simulink library "NFSModelsLibrary"  (R2020a)
settings: Solver=VariableStepAuto  StartTime=0.0  StopTime=10.0  RelTol=1e-3
undefined symbols (not defined in the file or in its folder): Earth, F, Light, MIL, Newton, nfs, Raphson, sigbuilder_block, WGS84
libraries: sharedutil x3, simulink x2, ModelsLibrary x2, $bdroot x2, aerolibwind2 x2, aerolibtransform2 x1
(part 2 of 3)

== system NFSModelsLibrary/3-AxisRateGyro/Noise Check/No Noise ==
  In : Inport
  Gain : Gain  Gain=0
  "Out " : Outport  VectorParamsAs1DForOutWhenUnconnected=off
  wires:
  Gain/1 -> "Out "/1
  In/1 -> Gain/1

== system NFSModelsLibrary/3-AxisRateGyro/Noise Check/Noisy Signal ==
  In : Inport
  "Out " : Outport  VectorParamsAs1DForOutWhenUnconnected=off
  wires:
  In/1 -> "Out "/1

== system NFSModelsLibrary/Aerodynamic Forces and Moments Derivatives/Forces/Aerodynamic Forces ==
  note: Since the forces and moments are in stability axis,
      | the beta has been multiplied with zero.
  CL : Inport  PortDimensions=1
  CD : Inport  Port=2  PortDimensions=1
  CY : Inport  Port=3  PortDimensions=1
  Dynamic Pressure : Inport  Port=4  PortDimensions=1
  Alpha : Inport  Port=5  PortDimensions=1
  Beta : Inport  Port=6  PortDimensions=1
  ChSign : Gain  Gain=-1  SaturateOnIntegerOverflow=on  OutDataTypeStr=Inherit: Same as input  ParamDataTypeStr=Inherit: Same as input
  ChSign1 : Gain  Gain=-1  SaturateOnIntegerOverflow=on  OutDataTypeStr=Inherit: Same as input  ParamDataTypeStr=Inherit: Same as input
  ChSign2 : Gain  Gain=0  SaturateOnIntegerOverflow=on  OutDataTypeStr=Inherit: Same as input  ParamDataTypeStr=Inherit: Same as input
  Mux : Mux  Inputs=3
  Product{,2..4} (4 alike) : Product  InputSameDT=on  SaturateOnIntegerOverflow=on  OutDataTypeStr=Inherit: Same as first input
  Product1 : Product  Multiplication=Matrix(*)  InputSameDT=on  SaturateOnIntegerOverflow=on  OutDataTypeStr=Inherit: Same as first input
  Wind2Body TM : Subsystem
  Wing Area : Constant  Value=nfs.refarea
  Aerodynamic Forces : Outport  PortDimensions=[3,1]  VectorParamsAs1DForOutWhenUnconnected=off
  wires:
  ChSign2/1 -> Wind2Body TM/2(Beta)
  Mux/1 -> Product1/2
  Product4/1 -> Mux/3
  Product3/1 -> Mux/2
  Product2/1 -> Mux/1
  ChSign1/1 -> Product4/2
  CY/1 -> Product3/2
  ChSign/1 -> Product2/2
  Product/1 -> Product4/1, Product3/1, Product2/1
  Wing Area/1 -> Product/2
  Dynamic Pressure/1 -> Product/1
  Alpha/1 -> Wind2Body TM/1(Alpha)
  CL/1 -> ChSign1/1
  CD/1 -> ChSign/1
  Beta/1 -> ChSign2/1
  Product1/1 -> Aerodynamic Forces/1
  Wind2Body TM/1(T_BW) -> Product1/1

== system NFSModelsLibrary/Aerodynamic Forces and Moments Derivatives/Forces/Force Coefficients Calculator ==
  Linear Velocity : Inport  PortDimensions=[3,1]
  Alpha : Inport  Port=2  PortDimensions=1
  Beta : Inport  Port=3
  Angular Velocity : Inport  Port=4  PortDimensions=[3,1]
  Control : Inport  Port=5  PortDimensions=[4,1]
  Alphadot : Inport  Port=6  PortDimensions=1
  Mach : Inport  Port=7
  Alpha2 : InportShadow  Port=2  PortDimensions=1
  Angular Velocity1 : InportShadow  Port=4  PortDimensions=[3,1]
  Control1 : InportShadow  Port=5  PortDimensions=[4,1]
  Demux1 : Demux  Outputs=3
      settings: DisplayOption=none
  Demux2 : Demux  Outputs=3
      settings: DisplayOption=none
  Demux3 : Demux
      settings: DisplayOption=none
  Demux4 : Demux
      settings: DisplayOption=none
  Drag Coefficient : Subsystem  mask{cD0=nfs.aero.cD0}
  Lift Coefficient : Subsystem  mask{cL0=nfs.aero.cL0, meanchord=nfs.meanchord}
      mask prompts: meanchord "Mean Aerodynamic Chord"
  Linear Velocity1 : InportShadow  PortDimensions=[3,1]
  Mach1 : InportShadow  Port=7
  SideForce Coefficient : Subsystem
  Terminator{,1..4} (5 alike) : Terminator
  CL : Outport  VectorParamsAs1DForOutWhenUnconnected=off
  CD : Outport  Port=2  VectorParamsAs1DForOutWhenUnconnected=off
  CY : Outport  Port=3  VectorParamsAs1DForOutWhenUnconnected=off
  wires:
  Linear Velocity1/1 -> SideForce Coefficient/1(Linear Velocity)
  Demux3/2 -> Lift Coefficient/4(DeltaFlap)
  Mach1/1 -> Drag Coefficient/7(Mach)
  Demux4/1 -> Drag Coefficient/3(DeltaElevator)
  Demux4/3 -> Drag Coefficient/5(DeltaAileron), SideForce Coefficient/5(DeltaAileron)
  Demux4/4 -> Drag Coefficient/6(DeltaRudder), SideForce Coefficient/6(DeltaRudder)
  Demux2/2 -> Terminator2/1
  Alpha/1 -> Lift Coefficient/2(Alpha)
  Demux3/3 -> Terminator3/1
  Demux3/4 -> Terminator4/1
  Demux1/2 -> Lift Coefficient/6(Q)
  Mach/1 -> Lift Coefficient/7(Mach)
  Demux4/2 -> Drag Coefficient/4(DeltaFlap)
  Angular Velocity/1 -> Demux1/1
  Control/1 -> Demux3/1
  Demux1/1 -> Terminator/1
  Beta/1 -> SideForce Coefficient/2(Beta)
  Angular Velocity1/1 -> Demux2/1
  Demux2/3 -> SideForce Coefficient/4(R)
  Control1/1 -> Demux4/1
  Demux3/1 -> Lift Coefficient/3(DeltaElevator)
  Demux2/1 -> SideForce Coefficient/3(P)
  Lift Coefficient/1(CL) -> Drag Coefficient/1(CL), CL/1
  Alphadot/1 -> Lift Coefficient/5(Alphadot)
  Demux1/3 -> Terminator1/1
  Alpha2/1 -> Drag Coefficient/2(alpha)
  Drag Coefficient/1(CD) -> CD/1
  SideForce Coefficient/1(CY) -> CY/1
  Linear Velocity/1 -> Lift Coefficient/1(Linear Velocity)

== system NFSModelsLibrary/Aerodynamic Forces and Moments Derivatives/Moments/Aerodynamic Moment  ==
  note: Since the forces and moments are in stability axis,
      | the beta has been multiplied with zero.
  Cl : Inport
  Cm : Inport  Port=2
  Cn : Inport  Port=3
  Dynamic Pressure : Inport  Port=4
  Alpha : Inport  Port=5  PortDimensions=1
  Beta : Inport  Port=6  PortDimensions=1
  Dynamic Pressure1 : InportShadow  Port=4
  Dynamic Pressure2 : InportShadow  Port=4
  Gain : Gain  Gain=0
  Mux : Mux  Inputs=3
  Pitch : Product  Inputs=4  InputSameDT=on  SaturateOnIntegerOverflow=on  OutDataTypeStr=Inherit: Same as first input
  Product1 : Product  Multiplication=Matrix(*)  InputSameDT=on  SaturateOnIntegerOverflow=on  OutDataTypeStr=Inherit: Same as first input
  Roll : Product  Inputs=4  InputSameDT=on  SaturateOnIntegerOverflow=on  OutDataTypeStr=Inherit: Same as first input
  Wind2Body TM : Subsystem
  Wing area : Constant  Value=nfs.refarea
  Wing chord : Constant  Value=nfs.meanchord
  Wing span : Constant  Value=nfs.span
  Wing span2 : Constant  Value=nfs.span
  Yaw : Product  Inputs=4  InputSameDT=on  SaturateOnIntegerOverflow=on  OutDataTypeStr=Inherit: Same as first input
  Aerodynamic Moments : Outport  PortDimensions=[3,1]  VectorParamsAs1DForOutWhenUnconnected=off
  wires:
  Gain/1 -> Wind2Body TM/2(Beta)
  Product1/1 -> Aerodynamic Moments/1
  Mux/1 -> Product1/2
  Alpha/1 -> Wind2Body TM/1(Alpha)
  Beta/1 -> Gain/1
  Wind2Body TM/1(T_BW) -> Product1/1
  Wing span/1 -> Roll/3
  Wing chord/1 -> Pitch/3
  Dynamic Pressure/1 -> Roll/1
  Cn/1 -> Yaw/4
  Cm/1 -> Pitch/4
  Cl/1 -> Roll/4
  Dynamic Pressure1/1 -> Pitch/1
  Dynamic Pressure2/1 -> Yaw/1
  Wing span2/1 -> Yaw/3
  Wing area/1 -> Pitch/2, Roll/2, Yaw/2
  Roll/1 -> Mux/1
  Pitch/1 -> Mux/2
  Yaw/1 -> Mux/3

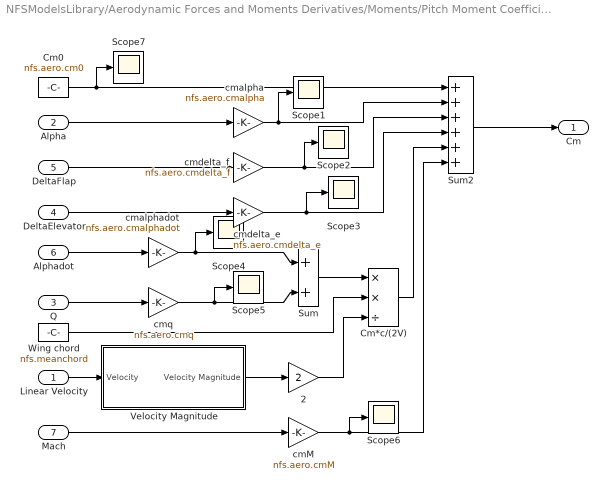
== system NFSModelsLibrary/Aerodynamic Forces and Moments Derivatives/Moments/Pitch Moment Coefficient ==
  Linear Velocity : Inport
  Alpha : Inport  Port=2
  Q : Inport  Port=3
  DeltaElevator : Inport  Port=4
  DeltaFlap : Inport  Port=5
  Alphadot : Inport  Port=6  PortDimensions=1
  Mach : Inport  Port=7  PortDimensions=1
  2 : Gain  Gain=2  SaturateOnIntegerOverflow=on  OutDataTypeStr=Inherit: Same as input  ParamDataTypeStr=Inherit: Same as input
  Cm*c/(2V) : Product  Inputs=**/  InputSameDT=on  SaturateOnIntegerOverflow=on  OutDataTypeStr=Inherit: Same as first input
  Cm0 : Constant  Value=nfs.aero.cm0
  Scope{1..7} (7 alike) : Scope
  Sum : Sum  InputSameDT=on  SaturateOnIntegerOverflow=on  OutDataTypeStr=Inherit: Same as first input
  Sum2 : Sum  Inputs=++++++  InputSameDT=on  SaturateOnIntegerOverflow=on  OutDataTypeStr=Inherit: Same as first input
  Velocity Magnitude : Subsystem
  Wing chord : Constant  Value=nfs.meanchord
  cmM : Gain  Gain=nfs.aero.cmM  SaturateOnIntegerOverflow=on  OutDataTypeStr=Inherit: Same as input  ParamDataTypeStr=Inherit: Same as input
  cmalpha : Gain  Gain=nfs.aero.cmalpha  SaturateOnIntegerOverflow=on  OutDataTypeStr=Inherit: Same as input  ParamDataTypeStr=Inherit: Same as input
  cmalphadot : Gain  Gain=nfs.aero.cmalphadot  SaturateOnIntegerOverflow=on  OutDataTypeStr=Inherit: Same as input  ParamDataTypeStr=Inherit: Same as input
  cmdelta_e : Gain  Gain=nfs.aero.cmdelta_e  SaturateOnIntegerOverflow=on  OutDataTypeStr=Inherit: Same as input  ParamDataTypeStr=Inherit: Same as input
  cmdelta_f : Gain  Gain=nfs.aero.cmdelta_f  SaturateOnIntegerOverflow=on  OutDataTypeStr=Inherit: Same as input  ParamDataTypeStr=Inherit: Same as input
  cmq : Gain  Gain=nfs.aero.cmq  SaturateOnIntegerOverflow=on  OutDataTypeStr=Inherit: Same as input  ParamDataTypeStr=Inherit: Same as input
  Cm : Outport  PortDimensions=1  VectorParamsAs1DForOutWhenUnconnected=off
  wires:
  Alphadot/1 -> cmalphadot/1
  2/1 -> Cm*c/(2V)/3
  Wing chord/1 -> Cm*c/(2V)/2
  cmq/1 -> Scope5/1, Sum/2
  cmalphadot/1 -> Scope4/1, Sum/1
  Sum/1 -> Cm*c/(2V)/1
  Cm0/1 -> Scope7/1, Sum2/1
  cmalpha/1 -> Scope1/1, Sum2/2
  cmdelta_f/1 -> Scope2/1, Sum2/3
  cmdelta_e/1 -> Scope3/1, Sum2/4
  Cm*c/(2V)/1 -> Sum2/5
  cmM/1 -> Scope6/1, Sum2/6
  Linear Velocity/1 -> Velocity Magnitude/1(Velocity)
  Velocity Magnitude/1(Velocity Magnitude) -> 2/1
  Alpha/1 -> cmalpha/1
  DeltaFlap/1 -> cmdelta_f/1
  DeltaElevator/1 -> cmdelta_e/1
  Q/1 -> cmq/1
  Mach/1 -> cmM/1
  Sum2/1 -> Cm/1

== system NFSModelsLibrary/Aerodynamic Forces and Moments Derivatives/Moments/Roll Moment Coefficient ==
  Linear Velocity : Inport
  Beta : Inport  Port=2  PortDimensions=1
  P : Inport  Port=3
  R : Inport  Port=4
  DeltaAileron : Inport  Port=5
  DeltaRudder : Inport  Port=6
  2 : Gain  Gain=2  SaturateOnIntegerOverflow=on  OutDataTypeStr=Inherit: Same as input  ParamDataTypeStr=Inherit: Same as input
  Cl*b/(2V) : Product  Inputs=**/  InputSameDT=on  SaturateOnIntegerOverflow=on  OutDataTypeStr=Inherit: Same as first input
  Sum : Sum  InputSameDT=on  SaturateOnIntegerOverflow=on  OutDataTypeStr=Inherit: Same as first input
  Sum2 : Sum  Inputs=++++  InputSameDT=on  SaturateOnIntegerOverflow=on  OutDataTypeStr=Inherit: Same as first input
  Velocity Magnitude : Subsystem
  Wing span : Constant  Value=nfs.span
  clbeta : Gain  Gain=nfs.aero.clbeta  SaturateOnIntegerOverflow=on  OutDataTypeStr=Inherit: Same as input  ParamDataTypeStr=Inherit: Same as input
  cldelta_a : Gain  Gain=nfs.aero.cldelta_a  SaturateOnIntegerOverflow=on  OutDataTypeStr=Inherit: Same as input  ParamDataTypeStr=Inherit: Same as input
  cldelta_r : Gain  Gain=nfs.aero.cldelta_r  SaturateOnIntegerOverflow=on  OutDataTypeStr=Inherit: Same as input  ParamDataTypeStr=Inherit: Same as input
  clp : Gain  Gain=nfs.aero.clp  SaturateOnIntegerOverflow=on  OutDataTypeStr=Inherit: Same as input  ParamDataTypeStr=Inherit: Same as input
  clr : Gain  Gain=nfs.aero.clr  SaturateOnIntegerOverflow=on  OutDataTypeStr=Inherit: Same as input  ParamDataTypeStr=Inherit: Same as input
  Cl : Outport  PortDimensions=1  VectorParamsAs1DForOutWhenUnconnected=off
  wires:
  clp/1 -> Sum/1
  clr/1 -> Sum/2
  Sum/1 -> Cl*b/(2V)/1
  Wing span/1 -> Cl*b/(2V)/2
  2/1 -> Cl*b/(2V)/3
  clbeta/1 -> Sum2/1
  cldelta_a/1 -> Sum2/2
  cldelta_r/1 -> Sum2/3
  Cl*b/(2V)/1 -> Sum2/4
  Linear Velocity/1 -> Velocity Magnitude/1(Velocity)
  Velocity Magnitude/1(Velocity Magnitude) -> 2/1
  Beta/1 -> clbeta/1
  DeltaAileron/1 -> cldelta_a/1
  DeltaRudder/1 -> cldelta_r/1
  P/1 -> clp/1
  R/1 -> clr/1
  Sum2/1 -> Cl/1

== system NFSModelsLibrary/Aerodynamic Forces and Moments Derivatives/Moments/Yaw Moment Coefficient ==
  Linear Velocity : Inport
  beta : Inport  Port=2  PortDimensions=1
  P : Inport  Port=3
  R : Inport  Port=4
  DeltaAileron : Inport  Port=5
  DeltaRudder : Inport  Port=6
  2 : Gain  Gain=2  SaturateOnIntegerOverflow=on  OutDataTypeStr=Inherit: Same as input  ParamDataTypeStr=Inherit: Same as input
  Cn*b/(2V) : Product  Inputs=**/  InputSameDT=on  SaturateOnIntegerOverflow=on  OutDataTypeStr=Inherit: Same as first input
  Sum : Sum  InputSameDT=on  SaturateOnIntegerOverflow=on  OutDataTypeStr=Inherit: Same as first input
  Sum2 : Sum  Inputs=++++  InputSameDT=on  SaturateOnIntegerOverflow=on  OutDataTypeStr=Inherit: Same as first input
  Velocity Magnitude : Subsystem
  Wing span : Constant  Value=nfs.span
  cnbeta : Gain  Gain=nfs.aero.cnbeta  SaturateOnIntegerOverflow=on  OutDataTypeStr=Inherit: Same as input  ParamDataTypeStr=Inherit: Same as input
  cndelta_a : Gain  Gain=nfs.aero.cndelta_a  SaturateOnIntegerOverflow=on  OutDataTypeStr=Inherit: Same as input  ParamDataTypeStr=Inherit: Same as input
  cndelta_r : Gain  Gain=nfs.aero.cndelta_r  SaturateOnIntegerOverflow=on  OutDataTypeStr=Inherit: Same as input  ParamDataTypeStr=Inherit: Same as input
  cnp : Gain  Gain=nfs.aero.cnp  SaturateOnIntegerOverflow=on  OutDataTypeStr=Inherit: Same as input  ParamDataTypeStr=Inherit: Same as input
  cnr : Gain  Gain=nfs.aero.cnr  SaturateOnIntegerOverflow=on  OutDataTypeStr=Inherit: Same as input  ParamDataTypeStr=Inherit: Same as input
  Cn : Outport  PortDimensions=1  VectorParamsAs1DForOutWhenUnconnected=off
  wires:
  Cn*b/(2V)/1 -> Sum2/4
  cndelta_r/1 -> Sum2/3
  cndelta_a/1 -> Sum2/2
  cnbeta/1 -> Sum2/1
  2/1 -> Cn*b/(2V)/3
  Wing span/1 -> Cn*b/(2V)/2
  Sum/1 -> Cn*b/(2V)/1
  cnr/1 -> Sum/2
  cnp/1 -> Sum/1
  Linear Velocity/1 -> Velocity Magnitude/1(Velocity)
  Velocity Magnitude/1(Velocity Magnitude) -> 2/1
  beta/1 -> cnbeta/1
  DeltaAileron/1 -> cndelta_a/1
  DeltaRudder/1 -> cndelta_r/1
  P/1 -> cnp/1
  R/1 -> cnr/1
  Sum2/1 -> Cn/1

== system NFSModelsLibrary/Aerodynamic Forces and Moments Derivatives/Turbulence/Turbulence Model ==
  In : Inport
  Dryden Turbulence Model : Subsystem  VariantControl=TurbulenceSelector == 1
  No Turbulence : Subsystem  VariantControl=TurbulenceSelector == 0
  Von-Karman Turbulence Model : Subsystem  VariantControl=TurbulenceSelector == 2
  Out : Outport  VectorParamsAs1DForOutWhenUnconnected=off

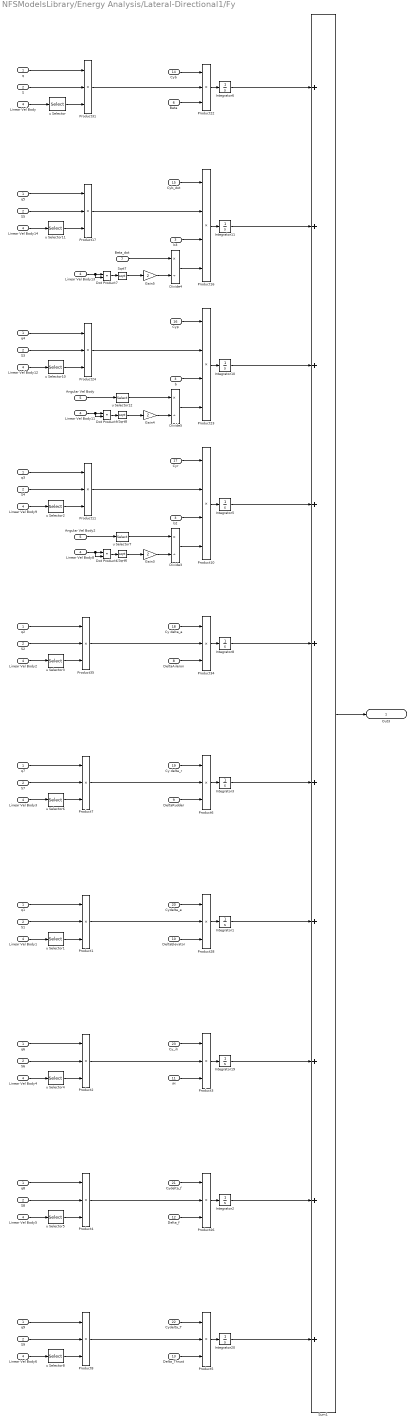
== system NFSModelsLibrary/Energy Analysis/Lateral-Directional1/Fy ==
  q : Inport
  S : Inport  Port=2
  b : Inport  Port=3
  Linear Vel Body : Inport  Port=4
  Angular Vel Body : Inport  Port=5
  Beta : Inport  Port=6
  Beta_dot : Inport  Port=7
  DeltaAileron : Inport  Port=8
  DeltaRudder : Inport  Port=9
  DeltaElevator : Inport  Port=10
  iH : Inport  Port=11
  Delta_f : Inport  Port=12
  Delta_Thrust : Inport  Port=13
  Cyb : Inport  Port=14
  Cyb_dot : Inport  Port=15
  Cyp : Inport  Port=16
  Cyr : Inport  Port=17
  Cy delta_a : Inport  Port=18
  Cy delta_r : Inport  Port=19
  Cydelta_e : Inport  Port=20
  Cydelta_f : Inport  Port=21
  Cydelta_T : Inport  Port=22
  Cy_ih : Inport  Port=23
  Angular Vel Body2 : InportShadow  Port=5
  Divide3 : Product  Inputs=*/
  Divide4 : Product  Inputs=*/
  Divide5 : Product  Inputs=*/
  Dot Product6 : DotProduct  InputSameDT=on  OutDataTypeStr=Inherit: Inherit via internal rule
  Dot Product7 : DotProduct  InputSameDT=on  OutDataTypeStr=Inherit: Inherit via internal rule
  Dot Product9 : DotProduct  InputSameDT=on  OutDataTypeStr=Inherit: Inherit via internal rule
  Gain3 : Gain  Gain=2
  Gain4 : Gain  Gain=2
  Gain5 : Gain  Gain=2
  Integrator{1..3,5..6,8,10..11,19..20} (10 alike) : Integrator
  Linear Vel Body{1..6,8..9,11..14} (12 alike) : InportShadow  Port=4
  Product{1..8,11,17,22,24,26,28,31,34..35} (17 alike) : Product  Inputs=3
  Product10 : Product  Inputs=4
  Product16 : Product  Inputs=4
  Product23 : Product  Inputs=4
  S{1..9} (9 alike) : InportShadow  Port=2
  Sqrt6 : Sqrt  SaturateOnIntegerOverflow=on
  Sqrt7 : Sqrt  SaturateOnIntegerOverflow=on
  Sqrt8 : Sqrt  SaturateOnIntegerOverflow=on
  Sum1 : Sum  Inputs=++++++++++
  b2 : InportShadow  Port=3
  b3 : InportShadow  Port=3
  q{1..9} (9 alike) : InportShadow
  u Selector{,1..6,8,10..11} (10 alike) : Selector  InputPortWidth=3  IndexOptions=Index vector (dialog)  Indices=[2]  OutputSizes=1
  u Selector12 : Selector  InputPortWidth=3  IndexOptions=Index vector (dialog)  Indices=[1]  OutputSizes=1
  u Selector7 : Selector  InputPortWidth=3  IndexOptions=Index vector (dialog)  Indices=[3]  OutputSizes=1
  Out3 : Outport  VectorParamsAs1DForOutWhenUnconnected=off
  wires:
  Integrator11/1 -> Sum1/2
  q/1 -> Product31/1
  S/1 -> Product31/2
  u Selector/1 -> Product31/3
  Linear Vel Body/1 -> u Selector/1
  Cy delta_a/1 -> Product34/1
  Product35/1 -> Product34/2
  DeltaAileron/1 -> Product34/3
  Product34/1 -> Integrator8/1
  Integrator8/1 -> Sum1/5
  Product24/1 -> Product23/2
  Divide5/1 -> Product23/4
  Product23/1 -> Integrator10/1
  q4/1 -> Product24/1
  S3/1 -> Product24/2
  u Selector10/1 -> Product24/3
  Linear Vel Body12/1 -> u Selector10/1
  Sqrt8/1 -> Gain4/1
  u Selector12/1 -> Divide5/1
  Dot Product9/1 -> Sqrt8/1
  Linear Vel Body11/1 -> Dot Product9/2, Dot Product9/1
  Angular Vel Body/1 -> u Selector12/1
  Cyp/1 -> Product23/1
  Sum1/1 -> Out3/1
  Cyb/1 -> Product22/1
  Product31/1 -> Product22/2
  Beta/1 -> Product22/3
  Product22/1 -> Integrator6/1
  Integrator6/1 -> Sum1/1
  b/1 -> Product23/3
  Gain4/1 -> Divide5/2
  Product11/1 -> Product10/2
  Divide3/1 -> Product10/4
  Product10/1 -> Integrator5/1
  q3/1 -> Product11/1
  S4/1 -> Product11/2
  u Selector2/1 -> Product11/3
  Linear Vel Body9/1 -> u Selector2/1
  Sqrt6/1 -> Gain3/1
  u Selector7/1 -> Divide3/1
  Dot Product6/1 -> Sqrt6/1
  Linear Vel Body8/1 -> Dot Product6/1, Dot Product6/2
  Angular Vel Body2/1 -> u Selector7/1
  Cyr/1 -> Product10/1
  b2/1 -> Product10/3
  Gain3/1 -> Divide3/2
  Integrator10/1 -> Sum1/3
  Integrator5/1 -> Sum1/4
  Product17/1 -> Product16/2
  Divide4/1 -> Product16/4
  Product16/1 -> Integrator11/1
  q5/1 -> Product17/1
  S5/1 -> Product17/2
  u Selector11/1 -> Product17/3
  Linear Vel Body14/1 -> u Selector11/1
  Sqrt7/1 -> Gain5/1
  Beta_dot/1 -> Divide4/1
  Dot Product7/1 -> Sqrt7/1
  Linear Vel Body13/1 -> Dot Product7/1, Dot Product7/2
  Cyb_dot/1 -> Product16/1
  b3/1 -> Product16/3
  Gain5/1 -> Divide4/2
  Cydelta_T/1 -> Product5/1
  Product8/1 -> Product5/2
  Delta_Thrust/1 -> Product5/3
  Product5/1 -> Integrator20/1
  Cydelta_f/1 -> Product26/1
  Product4/1 -> Product26/2
  Delta_f/1 -> Product26/3
  Product26/1 -> Integrator2/1
  Cydelta_e/1 -> Product28/1
  Product1/1 -> Product28/2
  DeltaElevator/1 -> Product28/3
  Product28/1 -> Integrator1/1
  Cy_ih/1 -> Product3/1
  Product2/1 -> Product3/2
  iH/1 -> Product3/3
  Product3/1 -> Integrator19/1
  q2/1 -> Product35/1
  S2/1 -> Product35/2
  u Selector3/1 -> Product35/3
  Linear Vel Body2/1 -> u Selector3/1
  Cy delta_r/1 -> Product6/1
  Product7/1 -> Product6/2
  DeltaRudder/1 -> Product6/3
  Product6/1 -> Integrator3/1
  q7/1 -> Product7/1
  S7/1 -> Product7/2
  u Selector6/1 -> Product7/3
  Linear Vel Body3/1 -> u Selector6/1
  Integrator3/1 -> Sum1/6
  Integrator1/1 -> Sum1/7
  Integrator19/1 -> Sum1/8
  Integrator2/1 -> Sum1/9
  Integrator20/1 -> Sum1/10
  q1/1 -> Product1/1
  S1/1 -> Product1/2
  u Selector1/1 -> Product1/3
  Linear Vel Body1/1 -> u Selector1/1
  q6/1 -> Product2/1
  S6/1 -> Product2/2
  u Selector4/1 -> Product2/3
  Linear Vel Body4/1 -> u Selector4/1
  q8/1 -> Product4/1
  S8/1 -> Product4/2
  u Selector5/1 -> Product4/3
  Linear Vel Body5/1 -> u Selector5/1
  q9/1 -> Product8/1
  S9/1 -> Product8/2
  u Selector8/1 -> Product8/3
  Linear Vel Body6/1 -> u Selector8/1

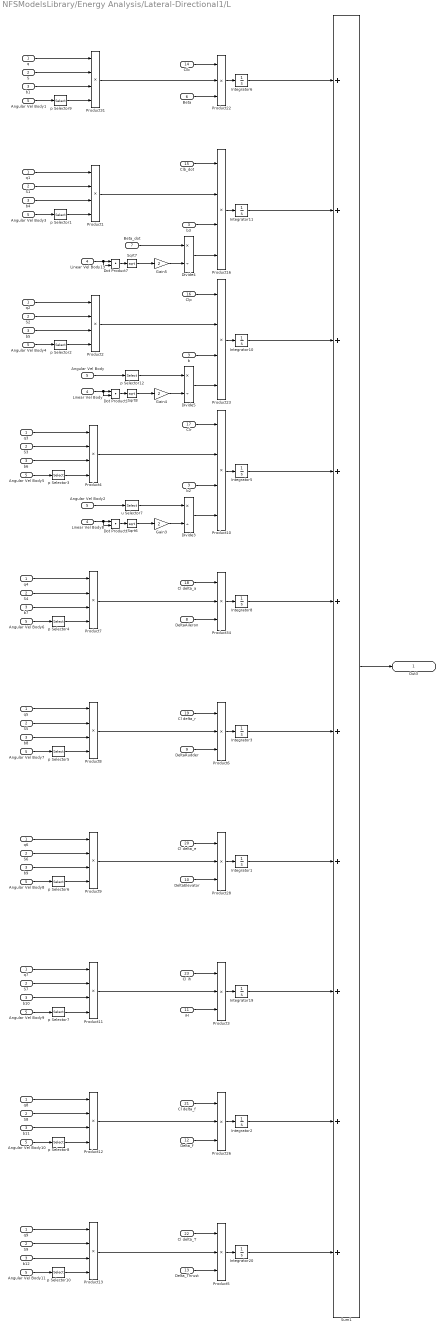
== system NFSModelsLibrary/Energy Analysis/Lateral-Directional1/L ==
  q : Inport
  S : Inport  Port=2
  b : Inport  Port=3
  Linear Vel Body : Inport  Port=4
  Angular Vel Body : Inport  Port=5
  Beta : Inport  Port=6
  Beta_dot : Inport  Port=7
  DeltaAileron : Inport  Port=8
  DeltaRudder : Inport  Port=9
  DeltaElevator : Inport  Port=10
  iH : Inport  Port=11
  Delta_f : Inport  Port=12
  Delta_Thrust : Inport  Port=13
  Clb : Inport  Port=14
  Clb_dot : Inport  Port=15
  Clp : Inport  Port=16
  Clr : Inport  Port=17
  Cl delta_a : Inport  Port=18
  Cl delta_r : Inport  Port=19
  Cl delta_e : Inport  Port=20
  Cl delta_f : Inport  Port=21
  Cl delta_T : Inport  Port=22
  Cl ih : Inport  Port=23
  Angular Vel Body{1..11} (11 alike) : InportShadow  Port=5
  Divide3 : Product  Inputs=*/
  Divide4 : Product  Inputs=*/
  Divide5 : Product  Inputs=*/
  Dot Product6 : DotProduct  InputSameDT=on  OutDataTypeStr=Inherit: Inherit via internal rule
  Dot Product7 : DotProduct  InputSameDT=on  OutDataTypeStr=Inherit: Inherit via internal rule
  Dot Product9 : DotProduct  InputSameDT=on  OutDataTypeStr=Inherit: Inherit via internal rule
  Gain3 : Gain  Gain=2
  Gain4 : Gain  Gain=2
  Gain5 : Gain  Gain=2
  Integrator{1..3,5..6,8,10..11,19..20} (10 alike) : Integrator
  Linear Vel Body13 : InportShadow  Port=4
  Linear Vel Body8 : InportShadow  Port=4
  Product{1..2,4,7..13,16,23,31} (13 alike) : Product  Inputs=4
  Product{3,5..6,22,26,28,34} (7 alike) : Product  Inputs=3
  S{1..9} (9 alike) : InportShadow  Port=2
  Sqrt6 : Sqrt  SaturateOnIntegerOverflow=on
  Sqrt7 : Sqrt  SaturateOnIntegerOverflow=on
  Sqrt8 : Sqrt  SaturateOnIntegerOverflow=on
  Sum1 : Sum  Inputs=++++++++++
  b{1..12} (12 alike) : InportShadow  Port=3
  p Selector{1..10,12} (11 alike) : Selector  InputPortWidth=3  IndexOptions=Index vector (dialog)  Indices=[1]  OutputSizes=1
  q{1..9} (9 alike) : InportShadow
  u Selector7 : Selector  InputPortWidth=3  IndexOptions=Index vector (dialog)  Indices=[3]  OutputSizes=1
  Out3 : Outport  VectorParamsAs1DForOutWhenUnconnected=off
  wires:
  Integrator11/1 -> Sum1/2
  q/1 -> Product31/1
  S/1 -> Product31/2
  p Selector9/1 -> Product31/4
  Cl delta_a/1 -> Product34/1
  Product7/1 -> Product34/2
  DeltaAileron/1 -> Product34/3
  Product34/1 -> Integrator8/1
  Integrator8/1 -> Sum1/5
  Product2/1 -> Product23/2
  Divide5/1 -> Product23/4
  Product23/1 -> Integrator10/1
  Sqrt8/1 -> Gain4/1
  p Selector12/1 -> Divide5/1
  Dot Product9/1 -> Sqrt8/1
  Linear Vel Body/1 -> Dot Product9/2, Dot Product9/1
  Angular Vel Body/1 -> p Selector12/1
  Clp/1 -> Product23/1
  Sum1/1 -> Out3/1
  Clb/1 -> Product22/1
  Product31/1 -> Product22/2
  Beta/1 -> Product22/3
  Product22/1 -> Integrator6/1
  Integrator6/1 -> Sum1/1
  b/1 -> Product23/3
  Gain4/1 -> Divide5/2
  Product4/1 -> Product10/2
  Divide3/1 -> Product10/4
  Product10/1 -> Integrator5/1
  Sqrt6/1 -> Gain3/1
  u Selector7/1 -> Divide3/1
  Dot Product6/1 -> Sqrt6/1
  Linear Vel Body8/1 -> Dot Product6/1, Dot Product6/2
  Angular Vel Body2/1 -> u Selector7/1
  Clr/1 -> Product10/1
  b2/1 -> Product10/3
  Gain3/1 -> Divide3/2
  Integrator10/1 -> Sum1/3
  Integrator5/1 -> Sum1/4
  Product1/1 -> Product16/2
  Divide4/1 -> Product16/4
  Product16/1 -> Integrator11/1
  Sqrt7/1 -> Gain5/1
  Beta_dot/1 -> Divide4/1
  Dot Product7/1 -> Sqrt7/1
  Linear Vel Body13/1 -> Dot Product7/1, Dot Product7/2
  Clb_dot/1 -> Product16/1
  b3/1 -> Product16/3
  Gain5/1 -> Divide4/2
  Cl delta_T/1 -> Product5/1
  Product13/1 -> Product5/2
  Delta_Thrust/1 -> Product5/3
  Product5/1 -> Integrator20/1
  Cl delta_f/1 -> Product26/1
  Product12/1 -> Product26/2
  Delta_f/1 -> Product26/3
  Product26/1 -> Integrator2/1
  Cl delta_e/1 -> Product28/1
  Product9/1 -> Product28/2
  DeltaElevator/1 -> Product28/3
  Product28/1 -> Integrator1/1
  Cl ih/1 -> Product3/1
  Product11/1 -> Product3/2
  iH/1 -> Product3/3
  Product3/1 -> Integrator19/1
  Cl delta_r/1 -> Product6/1
  Product8/1 -> Product6/2
  DeltaRudder/1 -> Product6/3
  Product6/1 -> Integrator3/1
  Integrator3/1 -> Sum1/6
  Integrator1/1 -> Sum1/7
  Integrator19/1 -> Sum1/8
  Integrator2/1 -> Sum1/9
  Integrator20/1 -> Sum1/10
  Angular Vel Body1/1 -> p Selector9/1
  b1/1 -> Product31/3
  q1/1 -> Product1/1
  S1/1 -> Product1/2
  p Selector1/1 -> Product1/4
  Angular Vel Body3/1 -> p Selector1/1
  b4/1 -> Product1/3
  q2/1 -> Product2/1
  S2/1 -> Product2/2
  p Selector2/1 -> Product2/4
  Angular Vel Body4/1 -> p Selector2/1
  b5/1 -> Product2/3
  q3/1 -> Product4/1
  S3/1 -> Product4/2
  p Selector3/1 -> Product4/4
  Angular Vel Body5/1 -> p Selector3/1
  b6/1 -> Product4/3
  q4/1 -> Product7/1
  S4/1 -> Product7/2
  p Selector4/1 -> Product7/4
  Angular Vel Body6/1 -> p Selector4/1
  b7/1 -> Product7/3
  q5/1 -> Product8/1
  S5/1 -> Product8/2
  p Selector5/1 -> Product8/4
  Angular Vel Body7/1 -> p Selector5/1
  b8/1 -> Product8/3
  q6/1 -> Product9/1
  S6/1 -> Product9/2
  p Selector6/1 -> Product9/4
  Angular Vel Body8/1 -> p Selector6/1
  b9/1 -> Product9/3
  q7/1 -> Product11/1
  S7/1 -> Product11/2
  p Selector7/1 -> Product11/4
  Angular Vel Body9/1 -> p Selector7/1
  b10/1 -> Product11/3
  q8/1 -> Product12/1
  S8/1 -> Product12/2
  p Selector8/1 -> Product12/4
  Angular Vel Body10/1 -> p Selector8/1
  b11/1 -> Product12/3
  q9/1 -> Product13/1
  S9/1 -> Product13/2
  p Selector10/1 -> Product13/4
  Angular Vel Body11/1 -> p Selector10/1
  b12/1 -> Product13/3

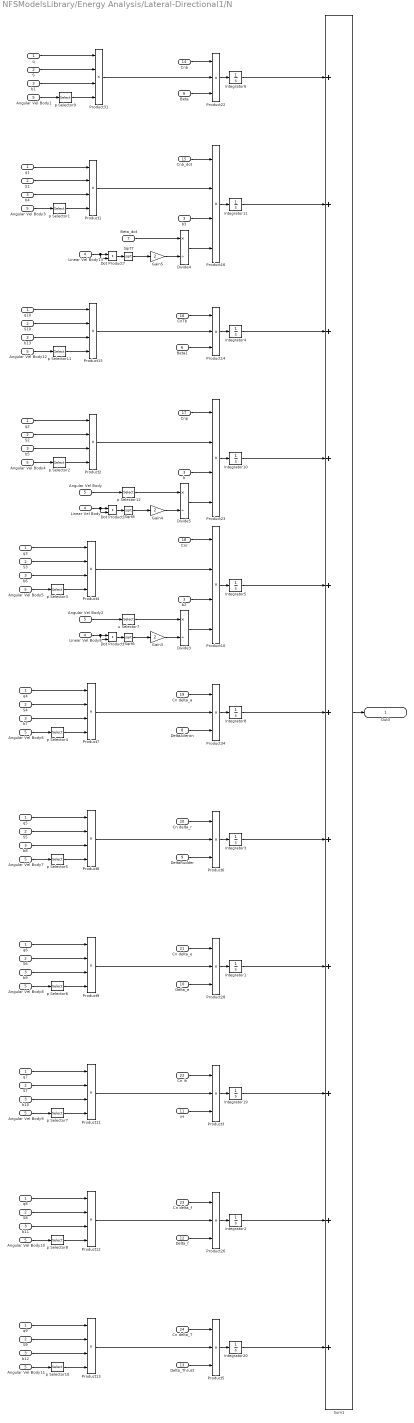
== system NFSModelsLibrary/Energy Analysis/Lateral-Directional1/N ==
  q : Inport
  S : Inport  Port=2
  b : Inport  Port=3
  Linear Vel Body : Inport  Port=4
  Angular Vel Body : Inport  Port=5
  Beta : Inport  Port=6
  Beta_dot : Inport  Port=7
  DeltaAileron : Inport  Port=8
  DeltaRudder : Inport  Port=9
  Delta_e : Inport  Port=10
  iH : Inport  Port=11
  Delta_f : Inport  Port=12
  Delta_Thrust : Inport  Port=13
  Cnb : Inport  Port=14
  Cnb_dot : Inport  Port=15
  CnTb : Inport  Port=16
  Cnp : Inport  Port=17
  Cnr : Inport  Port=18
  Cn delta_a : Inport  Port=19
  Cn delta_r : Inport  Port=20
  Cn delta_e : Inport  Port=21
  Cn ih : Inport  Port=22
  Cn delta_f : Inport  Port=23
  Cn delta_T : Inport  Port=24
  Angular Vel Body{1..12} (12 alike) : InportShadow  Port=5
  Beta1 : InportShadow  Port=6
  Divide3 : Product  Inputs=*/
  Divide4 : Product  Inputs=*/
  Divide5 : Product  Inputs=*/
  Dot Product6 : DotProduct  InputSameDT=on  OutDataTypeStr=Inherit: Inherit via internal rule
  Dot Product7 : DotProduct  InputSameDT=on  OutDataTypeStr=Inherit: Inherit via internal rule
  Dot Product9 : DotProduct  InputSameDT=on  OutDataTypeStr=Inherit: Inherit via internal rule
  Gain3 : Gain  Gain=2
  Gain4 : Gain  Gain=2
  Gain5 : Gain  Gain=2
  Integrator{1..6,8,10..11,19..20} (11 alike) : Integrator
  Linear Vel Body13 : InportShadow  Port=4
  Linear Vel Body8 : InportShadow  Port=4
  Product{1..2,4,7..13,15..16,23,31} (14 alike) : Product  Inputs=4
  Product{3,5..6,14,22,26,28,34} (8 alike) : Product  Inputs=3
  S{1..10} (10 alike) : InportShadow  Port=2
  Sqrt6 : Sqrt  SaturateOnIntegerOverflow=on
  Sqrt7 : Sqrt  SaturateOnIntegerOverflow=on
  Sqrt8 : Sqrt  SaturateOnIntegerOverflow=on
  Sum1 : Sum  Inputs=+++++++++++
  b{1..13} (13 alike) : InportShadow  Port=3
  p Selector{1..12} (12 alike) : Selector  InputPortWidth=3  IndexOptions=Index vector (dialog)  Indices=[1]  OutputSizes=1
  q{1..10} (10 alike) : InportShadow
  u Selector7 : Selector  InputPortWidth=3  IndexOptions=Index vector (dialog)  Indices=[3]  OutputSizes=1
  Out3 : Outport  VectorParamsAs1DForOutWhenUnconnected=off
  wires:
  Integrator11/1 -> Sum1/2
  q/1 -> Product31/1
  S/1 -> Product31/2
  p Selector9/1 -> Product31/4
  Cn delta_a/1 -> Product34/1
  Product7/1 -> Product34/2
  DeltaAileron/1 -> Product34/3
  Product34/1 -> Integrator8/1
  Product2/1 -> Product23/2
  Divide5/1 -> Product23/4
  Product23/1 -> Integrator10/1
  Sqrt8/1 -> Gain4/1
  p Selector12/1 -> Divide5/1
  Dot Product9/1 -> Sqrt8/1
  Linear Vel Body/1 -> Dot Product9/2, Dot Product9/1
  Angular Vel Body/1 -> p Selector12/1
  Cnp/1 -> Product23/1
  Cnb/1 -> Product22/1
  Product31/1 -> Product22/2
  Beta/1 -> Product22/3
  Product22/1 -> Integrator6/1
  Integrator6/1 -> Sum1/1
  b/1 -> Product23/3
  Gain4/1 -> Divide5/2
  Product4/1 -> Product10/2
  Divide3/1 -> Product10/4
  Product10/1 -> Integrator5/1
  Sqrt6/1 -> Gain3/1
  u Selector7/1 -> Divide3/1
  Dot Product6/1 -> Sqrt6/1
  Linear Vel Body8/1 -> Dot Product6/1, Dot Product6/2
  Angular Vel Body2/1 -> u Selector7/1
  Cnr/1 -> Product10/1
  b2/1 -> Product10/3
  Gain3/1 -> Divide3/2
  Product1/1 -> Product16/2
  Divide4/1 -> Product16/4
  Product16/1 -> Integrator11/1
  Sqrt7/1 -> Gain5/1
  Beta_dot/1 -> Divide4/1
  Dot Product7/1 -> Sqrt7/1
  Linear Vel Body13/1 -> Dot Product7/1, Dot Product7/2
  Cnb_dot/1 -> Product16/1
  b3/1 -> Product16/3
  Gain5/1 -> Divide4/2
  Cn delta_T/1 -> Product5/1
  Product13/1 -> Product5/2
  Delta_Thrust/1 -> Product5/3
  Product5/1 -> Integrator20/1
  Cn delta_f/1 -> Product26/1
  Product12/1 -> Product26/2
  Delta_f/1 -> Product26/3
  Product26/1 -> Integrator2/1
  Cn delta_e/1 -> Product28/1
  Product9/1 -> Product28/2
  Delta_e/1 -> Product28/3
  Product28/1 -> Integrator1/1
  Cn ih/1 -> Product3/1
  Product11/1 -> Product3/2
  iH/1 -> Product3/3
  Product3/1 -> Integrator19/1
  Cn delta_r/1 -> Product6/1
  Product8/1 -> Product6/2
  DeltaRudder/1 -> Product6/3
  Product6/1 -> Integrator3/1
  Angular Vel Body1/1 -> p Selector9/1
  b1/1 -> Product31/3
  q1/1 -> Product1/1
  S1/1 -> Product1/2
  p Selector1/1 -> Product1/4
  Angular Vel Body3/1 -> p Selector1/1
  b4/1 -> Product1/3
  q2/1 -> Product2/1
  S2/1 -> Product2/2
  p Selector2/1 -> Product2/4
  Angular Vel Body4/1 -> p Selector2/1
  b5/1 -> Product2/3
  q3/1 -> Product4/1
  S3/1 -> Product4/2
  p Selector3/1 -> Product4/4
  Angular Vel Body5/1 -> p Selector3/1
  b6/1 -> Product4/3
  q4/1 -> Product7/1
  S4/1 -> Product7/2
  p Selector4/1 -> Product7/4
  Angular Vel Body6/1 -> p Selector4/1
  b7/1 -> Product7/3
  q5/1 -> Product8/1
  S5/1 -> Product8/2
  p Selector5/1 -> Product8/4
  Angular Vel Body7/1 -> p Selector5/1
  b8/1 -> Product8/3
  q6/1 -> Product9/1
  S6/1 -> Product9/2
  p Selector6/1 -> Product9/4
  Angular Vel Body8/1 -> p Selector6/1
  b9/1 -> Product9/3
  q7/1 -> Product11/1
  S7/1 -> Product11/2
  p Selector7/1 -> Product11/4
  Angular Vel Body9/1 -> p Selector7/1
  b10/1 -> Product11/3
  q8/1 -> Product12/1
  S8/1 -> Product12/2
  p Selector8/1 -> Product12/4
  Angular Vel Body10/1 -> p Selector8/1
  b11/1 -> Product12/3
  q9/1 -> Product13/1
  S9/1 -> Product13/2
  p Selector10/1 -> Product13/4
  Angular Vel Body11/1 -> p Selector10/1
  b12/1 -> Product13/3
  q10/1 -> Product15/1
  S10/1 -> Product15/2
  p Selector11/1 -> Product15/4
  CnTb/1 -> Product14/1
  Product15/1 -> Product14/2
  Beta1/1 -> Product14/3
  Product14/1 -> Integrator4/1
  Angular Vel Body12/1 -> p Selector11/1
  b13/1 -> Product15/3
  Integrator20/1 -> Sum1/11
  Integrator2/1 -> Sum1/10
  Integrator19/1 -> Sum1/9
  Integrator1/1 -> Sum1/8
  Integrator3/1 -> Sum1/7
  Integrator8/1 -> Sum1/6
  Integrator5/1 -> Sum1/5
  Integrator10/1 -> Sum1/4
  Integrator4/1 -> Sum1/3
  Sum1/1 -> Out3/1

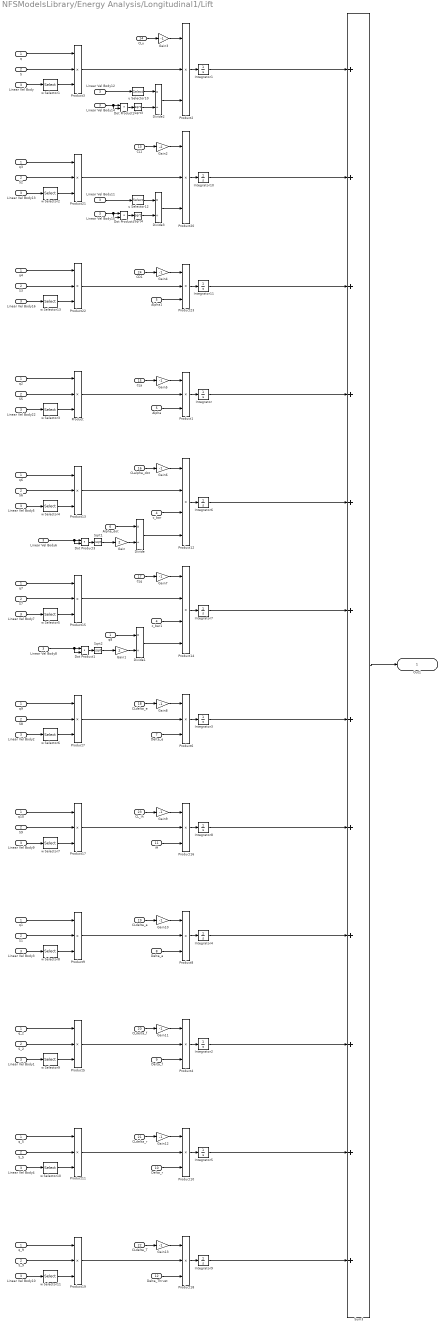
== system NFSModelsLibrary/Energy Analysis/Longitudinal1/Lift ==
  q : Inport
  S : Inport  Port=2
  Linear Vel Body : Inport  Port=3
  c_bar : Inport  Port=4
  Alpha : Inport  Port=5
  Alpha_dot : Inport  Port=6
  Delta_e : Inport  Port=7
  Delta_a : Inport  Port=8
  Delta_f : Inport  Port=9
  Delta_r : Inport  Port=10
  iH : Inport  Port=11
  Delta_Thrust : Inport  Port=12
  CL1 : Inport  Port=13
  CLu : Inport  Port=14
  CLa : Inport  Port=15
  CLalpha_dot : Inport  Port=16
  CLq : Inport  Port=17
  CLdelta_e : Inport  Port=18
  CLdelta_a : Inport  Port=19
  CLdelta_f : Inport  Port=20
  CLdelta_r : Inport  Port=21
  CLdelta_T : Inport  Port=22
  CL_ih : Inport  Port=23
  CD1 : Inport  Port=24
  Alpha1 : InportShadow  Port=5
  Divide{,1..3} (4 alike) : Product  Inputs=*/
  Dot Product{1..4} (4 alike) : DotProduct  InputSameDT=on  OutDataTypeStr=Inherit: Inherit via internal rule
  Gain : Gain  Gain=2
  Gain1 : Gain  Gain=2
  Gain{3..13} (11 alike) : Gain  Gain=-1
  Gain2 : Gain  Gain=-2
  Integrator{,1..11} (12 alike) : Integrator
  Linear Vel Body{1..16,22} (17 alike) : InportShadow  Port=3
  Product{,1..11,13,15..23} (22 alike) : Product  Inputs=3
  Product12 : Product  Inputs=4
  Product14 : Product  Inputs=4
  S{1..3,5..9} (8 alike) : InportShadow  Port=2
  S_2 : InportShadow  Port=2
  S_5 : InportShadow  Port=2
  S_9 : InportShadow  Port=2
  Sqrt{1..4} (4 alike) : Sqrt  SaturateOnIntegerOverflow=on
  Sum3 : Sum  Inputs=++++++++++++
  c_bar1 : InportShadow  Port=4
  q{1..4,6..10} (9 alike) : InportShadow
  q_2 : InportShadow
  q_5 : InportShadow
  q_9 : InportShadow
  u Selector10 : Selector  InputPortWidth=3  IndexOptions=Index vector (dialog)  Indices=[1]  OutputSizes=1
  u Selector12 : Selector  InputPortWidth=3  IndexOptions=Index vector (dialog)  Indices=[1]  OutputSizes=1
  w Selector{1..11,13} (12 alike) : Selector  InputPortWidth=3  IndexOptions=Index vector (dialog)  Indices=[3]  OutputSizes=1
  Out1 : Outport  VectorParamsAs1DForOutWhenUnconnected=off
  wires:
  Integrator1/1 -> Sum3/1
  CLu/1 -> Gain3/1
  Product3/1 -> Product2/2
  Divide2/1 -> Product2/3
  Product2/1 -> Integrator1/1
  Integrator10/1 -> Sum3/2
  q/1 -> Product3/1
  S/1 -> Product3/2
  Sum3/1 -> Out1/1
  w Selector1/1 -> Product3/3
  Linear Vel Body/1 -> w Selector1/1
  Sqrt3/1 -> Divide2/2
  u Selector10/1 -> Divide2/1
  Dot Product2/1 -> Sqrt3/1
  Linear Vel Body14/1 -> Dot Product2/1, Dot Product2/2
  Linear Vel Body12/1 -> u Selector10/1
  CL1/1 -> Gain2/1
  Product21/1 -> Product20/2
  Divide3/1 -> Product20/3
  Product20/1 -> Integrator10/1
  q3/1 -> Product21/1
  S2/1 -> Product21/2
  w Selector2/1 -> Product21/3
  Linear Vel Body13/1 -> w Selector2/1
  Sqrt4/1 -> Divide3/2
  u Selector12/1 -> Divide3/1
  Dot Product4/1 -> Sqrt4/1
  Linear Vel Body15/1 -> Dot Product4/2, Dot Product4/1
  Linear Vel Body11/1 -> u Selector12/1
  Gain2/1 -> Product20/1
  Integrator6/1 -> Sum3/5
  Integrator3/1 -> Sum3/7
  Integrator4/1 -> Sum3/9
  Integrator2/1 -> Sum3/10
  Integrator5/1 -> Sum3/11
  CLdelta_T/1 -> Gain13/1
  Product19/1 -> Product18/2
  Delta_Thrust/1 -> Product18/3
  Product18/1 -> Integrator9/1
  q_9/1 -> Product19/1
  S_9/1 -> Product19/2
  w Selector11/1 -> Product19/3
  Linear Vel Body10/1 -> w Selector11/1
  Integrator9/1 -> Sum3/12
  CLdelta_r/1 -> Gain12/1
  Product11/1 -> Product10/2
  Delta_r/1 -> Product10/3
  Product10/1 -> Integrator5/1
  q_5/1 -> Product11/1
  S_5/1 -> Product11/2
  w Selector10/1 -> Product11/3
  Linear Vel Body4/1 -> w Selector10/1
  CLdelta_f/1 -> Gain11/1
  Product5/1 -> Product4/2
  Delta_f/1 -> Product4/3
  Product4/1 -> Integrator2/1
  q_2/1 -> Product5/1
  S_2/1 -> Product5/2
  w Selector9/1 -> Product5/3
  Linear Vel Body1/1 -> w Selector9/1
  Alpha/1 -> Product1/3
  CLa/1 -> Gain5/1
  Product/1 -> Product1/2
  Product1/1 -> Integrator/1
  q2/1 -> Product/1
  S5/1 -> Product/2
  Linear Vel Body22/1 -> w Selector3/1
  w Selector3/1 -> Product/3
  CLdelta_e/1 -> Gain8/1
  Product7/1 -> Product6/2
  Delta_e/1 -> Product6/3
  Product6/1 -> Integrator3/1
  q9/1 -> Product7/1
  S8/1 -> Product7/2
  w Selector6/1 -> Product7/3
  Linear Vel Body2/1 -> w Selector6/1
  CLdelta_a/1 -> Gain10/1
  Product9/1 -> Product8/2
  Delta_a/1 -> Product8/3
  Product8/1 -> Integrator4/1
  q1/1 -> Product9/1
  S1/1 -> Product9/2
  w Selector8/1 -> Product9/3
  Linear Vel Body3/1 -> w Selector8/1
  CLalpha_dot/1 -> Gain6/1
  Product13/1 -> Product12/2
  c_bar/1 -> Product12/3
  Product12/1 -> Integrator6/1
  q6/1 -> Product13/1
  S6/1 -> Product13/2
  w Selector4/1 -> Product13/3
  Linear Vel Body5/1 -> w Selector4/1
  Gain/1 -> Divide/2
  Alpha_dot/1 -> Divide/1
  Divide/1 -> Product12/4
  Dot Product3/1 -> Sqrt1/1
  Linear Vel Body6/1 -> Dot Product3/1, Dot Product3/2
  Sqrt1/1 -> Gain/1
  CLq/1 -> Gain7/1
  Product15/1 -> Product14/2
  c_bar1/1 -> Product14/3
  Product14/1 -> Integrator7/1
  q7/1 -> Product15/1
  S7/1 -> Product15/2
  w Selector5/1 -> Product15/3
  Linear Vel Body7/1 -> w Selector5/1
  Gain1/1 -> Divide1/2
  q8/1 -> Divide1/1
  Divide1/1 -> Product14/4
  Dot Product1/1 -> Sqrt2/1
  Linear Vel Body8/1 -> Dot Product1/2, Dot Product1/1
  Sqrt2/1 -> Gain1/1
  CL_ih/1 -> Gain9/1
  Product17/1 -> Product16/2
  iH/1 -> Product16/3
  Product16/1 -> Integrator8/1
  q10/1 -> Product17/1
  S9/1 -> Product17/2
  w Selector7/1 -> Product17/3
  Linear Vel Body9/1 -> w Selector7/1
  Integrator8/1 -> Sum3/8
  Integrator/1 -> Sum3/4
  Integrator7/1 -> Sum3/6
  Alpha1/1 -> Product23/3
  CD1/1 -> Gain4/1
  Product22/1 -> Product23/2
  Product23/1 -> Integrator11/1
  q4/1 -> Product22/1
  S3/1 -> Product22/2
  Linear Vel Body16/1 -> w Selector13/1
  w Selector13/1 -> Product22/3
  Integrator11/1 -> Sum3/3
  Gain3/1 -> Product2/1
  Gain4/1 -> Product23/1
  Gain5/1 -> Product1/1
  Gain6/1 -> Product12/1
  Gain7/1 -> Product14/1
  Gain8/1 -> Product6/1
  Gain9/1 -> Product16/1
  Gain10/1 -> Product8/1
  Gain11/1 -> Product4/1
  Gain12/1 -> Product10/1
  Gain13/1 -> Product18/1

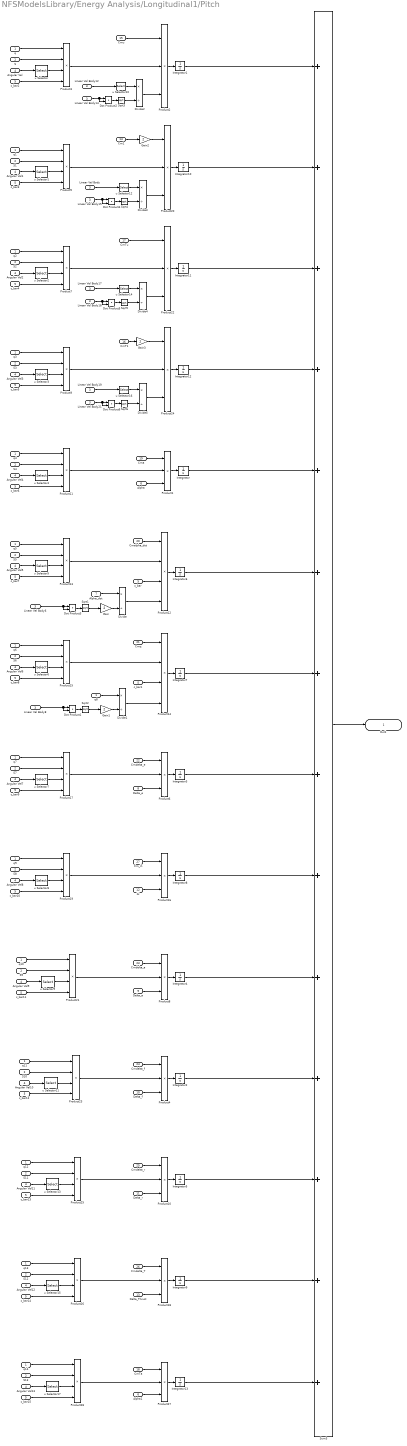
== system NFSModelsLibrary/Energy Analysis/Longitudinal1/Pitch ==
  q : Inport
  S : Inport  Port=2
  Linear Vel Body : Inport  Port=3
  Angular Vel : Inport  Port=4
  c_bar : Inport  Port=5
  Alpha : Inport  Port=6
  Alpha_dot : Inport  Port=7
  Delta_e : Inport  Port=8
  Delta_a : Inport  Port=9
  Delta_f : Inport  Port=10
  Delta_r : Inport  Port=11
  iH : Inport  Port=12
  Delta_Thrust : Inport  Port=13
  Cm1 : Inport  Port=14
  Cmu : Inport  Port=15
  CmT1 : Inport  Port=16
  CmTu : Inport  Port=17
  CmTa : Inport  Port=18
  Cma : Inport  Port=19
  Cmalpha_dot : Inport  Port=20
  Cmq : Inport  Port=21
  Cmdelta_e : Inport  Port=22
  Cmdelta_a : Inport  Port=23
  Cmdelta_f : Inport  Port=24
  Cmdelta_r : Inport  Port=25
  Cmdelta_T : Inport  Port=26
  Cm_ih : Inport  Port=27
  Alpha1 : InportShadow  Port=6
  Angular Vel{1..13} (13 alike) : InportShadow  Port=4
  Divide{,1..5} (6 alike) : Product  Inputs=*/
  Dot Product{1..6} (6 alike) : DotProduct  InputSameDT=on  OutDataTypeStr=Inherit: Inherit via internal rule
  Gain{,1..3} (4 alike) : Gain  Gain=2
  Integrator{,1..13} (14 alike) : Integrator
  Linear Vel Body{6,8,12,14..15,17..19,21} (9 alike) : InportShadow  Port=3
  Product{1..2,4,6,8,10,16,18,20,22,24,27} (12 alike) : Product  Inputs=3
  Product{3,5,7,9,11..15,17,19,21,23,25..26,28} (16 alike) : Product  Inputs=4
  S{1..13} (13 alike) : InportShadow  Port=2
  Sqrt{1..6} (6 alike) : Sqrt  SaturateOnIntegerOverflow=on
  Sum3 : Sum  Inputs=++++++++++++++
  c_bar{1..15} (15 alike) : InportShadow  Port=5
  q{1..14} (14 alike) : InportShadow
  u Selector{,1..9,11,13,15,17} (14 alike) : Selector  InputPortWidth=3  IndexOptions=Index vector (dialog)  Indices=[2]  OutputSizes=1
  u Selector{10,12,14,16} (4 alike) : Selector  InputPortWidth=3  IndexOptions=Index vector (dialog)  Indices=[1]  OutputSizes=1
  Out1 : Outport  VectorParamsAs1DForOutWhenUnconnected=off
  wires:
  Integrator7/1 -> Sum3/7
  Integrator12/1 -> Sum3/4
  Gain3/1 -> Product24/1
  Linear Vel Body19/1 -> u Selector16/1
  Linear Vel Body21/1 -> Dot Product6/1, Dot Product6/2
  Dot Product6/1 -> Sqrt6/1
  u Selector16/1 -> Divide5/1
  Sqrt6/1 -> Divide5/2
  Product24/1 -> Integrator12/1
  Divide5/1 -> Product24/3
  Product9/1 -> Product24/2
  CmT1/1 -> Gain3/1
  Integrator11/1 -> Sum3/3
  Linear Vel Body17/1 -> u Selector14/1
  Linear Vel Body18/1 -> Dot Product5/2, Dot Product5/1
  Dot Product5/1 -> Sqrt5/1
  u Selector14/1 -> Divide4/1
  Sqrt5/1 -> Divide4/2
  Product22/1 -> Integrator11/1
  Divide4/1 -> Product22/3
  Product7/1 -> Product22/2
  CmTu/1 -> Product22/1
  Gain2/1 -> Product20/1
  Linear Vel Body/1 -> u Selector12/1
  Linear Vel Body15/1 -> Dot Product4/1, Dot Product4/2
  Dot Product4/1 -> Sqrt4/1
  u Selector12/1 -> Divide3/1
  Sqrt4/1 -> Divide3/2
  Product20/1 -> Integrator10/1
  Divide3/1 -> Product20/3
  Product5/1 -> Product20/2
  Cm1/1 -> Gain2/1
  Integrator/1 -> Sum3/5
  Integrator8/1 -> Sum3/9
  Product16/1 -> Integrator8/1
  iH/1 -> Product16/3
  Product19/1 -> Product16/2
  Cm_ih/1 -> Product16/1
  Sqrt2/1 -> Gain1/1
  Linear Vel Body8/1 -> Dot Product1/1, Dot Product1/2
  Dot Product1/1 -> Sqrt2/1
  Divide1/1 -> Product14/4
  q8/1 -> Divide1/1
  Gain1/1 -> Divide1/2
  Product14/1 -> Integrator7/1
  c_bar1/1 -> Product14/3
  Product15/1 -> Product14/2
  Cmq/1 -> Product14/1
  Sqrt1/1 -> Gain/1
  Linear Vel Body6/1 -> Dot Product3/2, Dot Product3/1
  Dot Product3/1 -> Sqrt1/1
  Divide/1 -> Product12/4
  Alpha_dot/1 -> Divide/1
  Gain/1 -> Divide/2
  Product12/1 -> Integrator6/1
  c_bar/1 -> Product12/3
  Product13/1 -> Product12/2
  Cmalpha_dot/1 -> Product12/1
  Product8/1 -> Integrator4/1
  Delta_a/1 -> Product8/3
  Product21/1 -> Product8/2
  Cmdelta_a/1 -> Product8/1
  Product6/1 -> Integrator3/1
  Delta_e/1 -> Product6/3
  Product17/1 -> Product6/2
  Cmdelta_e/1 -> Product6/1
  Product1/1 -> Integrator/1
  Product11/1 -> Product1/2
  Cma/1 -> Product1/1
  Alpha/1 -> Product1/3
  Product4/1 -> Integrator2/1
  Delta_f/1 -> Product4/3
  Product23/1 -> Product4/2
  Cmdelta_f/1 -> Product4/1
  Product10/1 -> Integrator5/1
  Delta_r/1 -> Product10/3
  Product25/1 -> Product10/2
  Cmdelta_r/1 -> Product10/1
  Integrator9/1 -> Sum3/13
  Product18/1 -> Integrator9/1
  Delta_Thrust/1 -> Product18/3
  Product26/1 -> Product18/2
  Cmdelta_T/1 -> Product18/1
  Integrator5/1 -> Sum3/12
  Integrator2/1 -> Sum3/11
  Integrator4/1 -> Sum3/10
  Integrator3/1 -> Sum3/8
  Integrator6/1 -> Sum3/6
  Linear Vel Body12/1 -> u Selector10/1
  Linear Vel Body14/1 -> Dot Product2/2, Dot Product2/1
  Dot Product2/1 -> Sqrt3/1
  u Selector10/1 -> Divide2/1
  Sqrt3/1 -> Divide2/2
  Angular Vel/1 -> u Selector/1
  u Selector/1 -> Product3/3
  Sum3/1 -> Out1/1
  S/1 -> Product3/2
  q/1 -> Product3/1
  Integrator10/1 -> Sum3/2
  Product2/1 -> Integrator1/1
  Divide2/1 -> Product2/3
  Product3/1 -> Product2/2
  Integrator1/1 -> Sum3/1
  CmTa/1 -> Product27/1
  Product28/1 -> Product27/2
  Product27/1 -> Integrator13/1
  Alpha1/1 -> Product27/3
  Integrator13/1 -> Sum3/14
  c_bar2/1 -> Product3/4
  Angular Vel1/1 -> u Selector1/1
  u Selector1/1 -> Product5/3
  S1/1 -> Product5/2
  q1/1 -> Product5/1
  c_bar3/1 -> Product5/4
  Angular Vel2/1 -> u Selector2/1
  u Selector2/1 -> Product7/3
  S2/1 -> Product7/2
  q2/1 -> Product7/1
  c_bar4/1 -> Product7/4
  Angular Vel3/1 -> u Selector3/1
  u Selector3/1 -> Product9/3
  S3/1 -> Product9/2
  q3/1 -> Product9/1
  c_bar5/1 -> Product9/4
  Angular Vel4/1 -> u Selector4/1
  u Selector4/1 -> Product11/3
  S4/1 -> Product11/2
  q4/1 -> Product11/1
  c_bar6/1 -> Product11/4
  Angular Vel5/1 -> u Selector5/1
  u Selector5/1 -> Product13/3
  S5/1 -> Product13/2
  q5/1 -> Product13/1
  c_bar7/1 -> Product13/4
  Angular Vel6/1 -> u Selector6/1
  u Selector6/1 -> Product15/3
  S6/1 -> Product15/2
  q6/1 -> Product15/1
  c_bar8/1 -> Product15/4
  Angular Vel7/1 -> u Selector7/1
  u Selector7/1 -> Product17/3
  S7/1 -> Product17/2
  q7/1 -> Product17/1
  c_bar9/1 -> Product17/4
  Angular Vel8/1 -> u Selector8/1
  u Selector8/1 -> Product19/3
  S8/1 -> Product19/2
  q9/1 -> Product19/1
  c_bar10/1 -> Product19/4
  Angular Vel9/1 -> u Selector9/1
  u Selector9/1 -> Product21/3
  S9/1 -> Product21/2
  q10/1 -> Product21/1
  c_bar11/1 -> Product21/4
  Angular Vel10/1 -> u Selector11/1
  u Selector11/1 -> Product23/3
  S10/1 -> Product23/2
  q11/1 -> Product23/1
  c_bar12/1 -> Product23/4
  Angular Vel11/1 -> u Selector13/1
  u Selector13/1 -> Product25/3
  S11/1 -> Product25/2
  q12/1 -> Product25/1
  c_bar13/1 -> Product25/4
  Angular Vel12/1 -> u Selector15/1
  u Selector15/1 -> Product26/3
  S12/1 -> Product26/2
  q13/1 -> Product26/1
  c_bar14/1 -> Product26/4
  Angular Vel13/1 -> u Selector17/1
  u Selector17/1 -> Product28/3
  S13/1 -> Product28/2
  q14/1 -> Product28/1
  c_bar15/1 -> Product28/4
  Cmu/1 -> Product2/1
